simulink model "sampleModel1511"  (R2023a)
settings: Solver=VariableStepAuto  StartTime=0.0  StopTime=10.0  RelTol=1e-3
libraries: hdlsllib x6, simulink x4
settings Model: Creator=user1  LastModifiedBy=user1

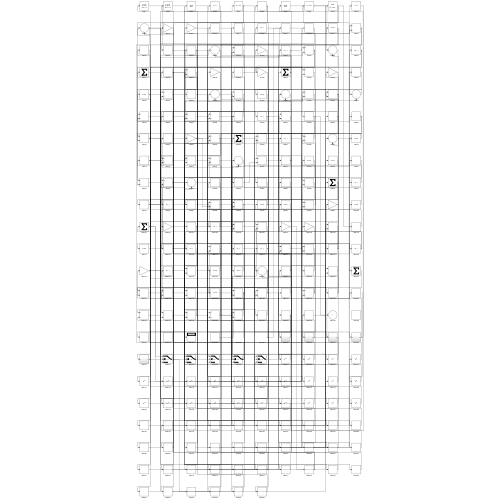
[thumbnail: Simulink's stored preview of the top-level diagram]
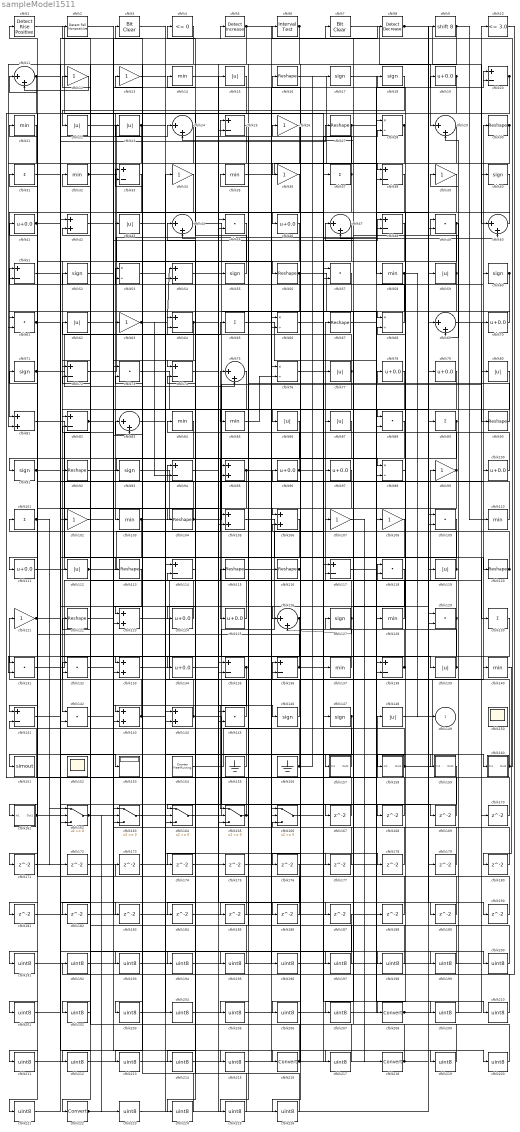
== system sampleModel1511 ==
  cfblk1 : hdlsllib/Logic and Bit Operations/Detect Rise Positive  vinit=0  OutDataTypeStr=boolean
  cfblk10 : hdlsllib/Logic and Bit Operations/Compare To Constant  relop=<=  const=3.0  OutDataTypeStr=boolean
  cfblk{19,41,46,70,78..79,96..97,100,111,124..125,134} (13 alike) : Bias  Bias=0.0  SaturateOnIntegerOverflow=off
  cfblk{31,37,65,89,101,130} (6 alike) : Sum  Inputs=+
  cfblk{12..13,26,34,36,39,63,99,102,107..108,121} (12 alike) : Gain
  cfblk{14,21,32,35,58,84..85,103,110,128,137,140} (12 alike) : MinMax
  cfblk{16,27,30,56,67,90,92,104,113,115..116,120,122} (13 alike) : Reshape
  cfblk{42,54,81,95,105..106,123,133,143..144} (10 alike) : Sum
  cfblk{45,49,57,61,73,88,109,118,129,131..132,142,145} (13 alike) : DotProduct  OutDataTypeStr=Inherit: Inherit via internal rule
  cfblk{11,24,29,44,47,50,69,75,83,126} (10 alike) : Sum  Inputs=|++
  cfblk{15,22..23,43,59,62,77,80,86..87,112,119,139,148} (14 alike) : Abs  SaturateOnIntegerOverflow=off
  cfblk{20,25,33,38,48,51,64,72,74,82,94,114,117,135..136,138,141} (17 alike) : Sum  Inputs=+-
  cfblk{17..18,40,52,55,60,71,91,93,127,146..147} (12 alike) : Signum
  cfblk150 : Scope
      settings: Floating=on
  cfblk151 : ToWorkspace  VariableName=simout  SaveFormat=Timeseries  SampleTime=-1
  cfblk152 : Scope
      settings: Floating=on
  cfblk153 : Display
  cfblk154 : hdlsllib/Sources/Counter Free-Running  NumBits=16  tsamp=-1
  cfblk155 : Ground
  cfblk156 : Ground
  cfblk157 : Subsystem
      settings: LibrarySourceBlock=|
      | hdlsllib/Ports &
      | Subsystems/Subsystem
  cfblk158 : Subsystem
      settings: LibrarySourceBlock=|
      | hdlsllib/Ports &
      | Subsystems/Subsystem
  cfblk159 : Subsystem
      settings: LibrarySourceBlock=|
      | hdlsllib/Ports &
      | Subsystems/Subsystem
  cfblk160 : Subsystem
      settings: LibrarySourceBlock=|
      | hdlsllib/Ports &
      | Subsystems/Subsystem
  cfblk161 : Subsystem
      settings: LibrarySourceBlock=|
      | hdlsllib/Ports &
      | Subsystems/Subsystem
  cfblk{162..166} (5 alike) : Switch  SaturateOnIntegerOverflow=off  InputSameDT=off
  cfblk{167..190} (24 alike) : Delay  SampleTime=1
  cfblk{191..207,209..215,217,219..221,223..226} (32 alike) : DataTypeConversion  OutDataTypeStr=uint8  SaturateOnIntegerOverflow=off  RndMeth=Floor
  cfblk2 : hdlsllib/Logic and Bit Operations/Detect Fall Nonpositive  vinit=0  OutDataTypeStr=boolean
  cfblk{208,216,218,222} (4 alike) : DataTypeConversion  SaturateOnIntegerOverflow=off  RndMeth=Floor
  cfblk{28,53,66,68,76,98} (6 alike) : Product  Inputs=*/  RndMeth=Zero  SaturateOnIntegerOverflow=on
  cfblk3 : simulink/Logic and Bit Operations/Bit Clear  iBit=0
      settings: LibrarySourceBlock=|
      | hdlsllib/Logic and Bit
      | Operations/Bit Clear
  cfblk4 : hdlsllib/Logic and Bit Operations/Compare To Zero  relop=<=  OutDataTypeStr=boolean
  cfblk5 : simulink/Logic and Bit Operations/Detect Increase  vinit=0.0  OutDataTypeStr=boolean
      settings: LibrarySourceBlock=|
      | hdlsllib/Logic and Bit
      | Operations/Detect
      | Increase
  cfblk6 : hdlsllib/Logic and Bit Operations/Interval Test  IntervalClosedRight=on  uplimit=0.5  IntervalClosedLeft=on  lowlimit=-0.5  OutDataTypeStr=boolean
  cfblk7 : simulink/Logic and Bit Operations/Bit Clear  iBit=0
      settings: LibrarySourceBlock=|
      | hdlsllib/Logic and Bit
      | Operations/Bit Clear
  cfblk8 : simulink/Logic and Bit Operations/Detect Decrease  vinit=0.0  OutDataTypeStr=boolean
      settings: LibrarySourceBlock=|
      | hdlsllib/Logic and Bit
      | Operations/Detect
      | Decrease
  cfblk9 : ArithShift  BitShiftNumber=8
  cfblk149 : Outport  VectorParamsAs1DForOutWhenUnconnected=off
  wires:
  cfblk20/1 -> cfblk103/1, cfblk164/3
  cfblk44/1 -> cfblk139/1
  cfblk18/1 -> cfblk22/1
  cfblk19/1 -> cfblk74/1, cfblk181/1
  cfblk33/1 -> cfblk81/1
  cfblk92/1 -> cfblk98/1
  cfblk87/1 -> cfblk125/1
  cfblk158/1(Out1) -> cfblk30/1, cfblk72/2
  cfblk65/1 -> cfblk138/1
  cfblk107/1 -> cfblk218/1
  cfblk26/1 -> cfblk91/1
  cfblk128/1 -> cfblk67/1
  cfblk32/1 -> cfblk56/1, cfblk72/1, cfblk215/1
  cfblk78/1 -> cfblk88/1
  cfblk123/1 -> cfblk136/1
  cfblk59/1 -> cfblk141/1, cfblk24/2, cfblk165/3
  cfblk157/1(Out1) -> cfblk83/1
  cfblk55/1 -> cfblk4/1
  cfblk84/1 -> cfblk133/1
  cfblk75/1 -> cfblk142/1
  cfblk160/1(Out1) -> cfblk6/1, cfblk33/1
  cfblk63/1 -> cfblk54/1, cfblk94/2
  cfblk15/1 -> cfblk143/1
  cfblk11/1 -> cfblk148/1, cfblk129/2, cfblk189/1
  cfblk71/1 -> cfblk64/1, cfblk75/2
  cfblk47/1 -> cfblk82/1
  cfblk159/1(Out1) -> cfblk164/1
  cfblk161/1(Out1) -> cfblk51/2, cfblk183/1
  cfblk37/1 -> cfblk14/1, cfblk162/2
  cfblk126/1 -> cfblk131/2, cfblk185/1
  cfblk60/1 -> cfblk157/1(In1), cfblk145/2
  cfblk80/1 -> cfblk158/1(In1)
  cfblk72/1 -> cfblk48/1
  cfblk46/1 -> cfblk123/1
  cfblk103/1 -> cfblk9/1, cfblk182/1
  cfblk38/1 -> cfblk106/1
  cfblk112/1 -> cfblk75/1, cfblk8/1
  cfblk85/1 -> cfblk76/2
  cfblk91/1 -> cfblk27/1, cfblk5/1, cfblk217/1
  cfblk62/1 -> cfblk216/1
  cfblk89/1 -> cfblk104/1, cfblk207/1
  cfblk129/1 -> cfblk74/2, cfblk174/1
  cfblk148/1 -> cfblk89/1
  cfblk164/1 -> cfblk37/1
  cfblk77/1 -> cfblk32/1, cfblk163/3
  cfblk23/1 -> cfblk43/1, cfblk177/1
  cfblk22/1 -> cfblk77/1
  cfblk16/1 -> cfblk58/1
  cfblk41/1 -> cfblk161/1(In1), cfblk135/2
  cfblk119/1 -> cfblk7/1, cfblk47/2
  cfblk50/1 -> cfblk46/1
  cfblk111/1 -> cfblk64/2
  cfblk35/1 -> cfblk38/1
  cfblk96/1 -> cfblk84/1, cfblk50/2
  cfblk134/1 -> cfblk15/1
  cfblk141/1 -> cfblk100/1
  cfblk110/1 -> cfblk41/1
  cfblk70/1 -> cfblk68/1
  cfblk156/1 -> cfblk94/1, cfblk17/1
  cfblk133/1 -> cfblk99/1
  cfblk136/1 -> cfblk51/1, cfblk168/1
  cfblk25/1 -> cfblk144/2
  cfblk101/1 -> cfblk162/1, cfblk172/1
  cfblk79/1 -> cfblk133/2
  cfblk146/1 -> cfblk35/1
  cfblk14/1 -> cfblk126/1
  cfblk40/1 -> cfblk44/2
  cfblk4/1 -> cfblk81/2
  cfblk143/1 -> cfblk121/1, cfblk178/1
  cfblk154/1 -> cfblk116/1
  cfblk56/1 -> cfblk128/1, cfblk134/1
  cfblk144/1 -> cfblk118/1, cfblk166/2, cfblk132/1
  cfblk3/1 -> cfblk120/1
  cfblk98/1 -> cfblk78/1
  cfblk127/1 -> cfblk126/2, cfblk12/1, cfblk3/1
  cfblk39/1 -> cfblk208/1
  cfblk116/1 -> cfblk96/1, cfblk226/1
  cfblk1/1 -> cfblk117/1
  cfblk49/1 -> cfblk112/1, cfblk69/2
  cfblk86/1 -> cfblk151/1
  cfblk125/1 -> cfblk73/2
  cfblk142/1 -> cfblk65/1
  cfblk105/1 -> cfblk147/1
  cfblk58/1 -> cfblk124/1, cfblk149/1
  cfblk131/1 -> cfblk80/1
  cfblk81/1 -> cfblk130/1
  cfblk97/1 -> cfblk113/1
  cfblk165/1 -> cfblk2/1, cfblk105/1
  cfblk29/1 -> cfblk36/1
  cfblk104/1 -> cfblk40/1, cfblk33/2
  cfblk166/1 -> cfblk137/1
  cfblk155/1 -> cfblk71/1
  cfblk64/1 -> cfblk123/2, cfblk146/1
  cfblk24/1 -> cfblk61/1
  cfblk36/1 -> cfblk54/2
  cfblk135/1 -> cfblk165/1, cfblk163/2
  cfblk163/1 -> cfblk140/1
  cfblk68/1 -> cfblk21/1
  cfblk139/1 -> cfblk18/1, cfblk29/2
  cfblk99/1 -> cfblk68/2, cfblk184/1
  cfblk9/1 -> cfblk86/1, cfblk110/1, cfblk162/3
  cfblk73/1 -> cfblk119/1
  cfblk76/1 -> cfblk28/2
  cfblk30/1 -> cfblk186/1, cfblk214/1
  cfblk120/1 -> cfblk49/1, cfblk31/1
  cfblk6/1 -> cfblk165/2, cfblk195/1
  cfblk54/1 -> cfblk118/2
  cfblk5/1 -> cfblk63/1, cfblk159/1(In1), cfblk202/1
  cfblk138/1 -> cfblk26/1, cfblk131/1
  cfblk95/1 -> cfblk20/2, cfblk211/1
  cfblk121/1 -> cfblk136/2, cfblk24/1
  cfblk106/1 -> cfblk142/2
  cfblk93/1 -> cfblk97/1
  cfblk61/1 -> cfblk105/2, cfblk193/1
  cfblk113/1 -> cfblk143/2
  cfblk124/1 -> cfblk52/1
  cfblk28/1 -> cfblk92/1, cfblk221/1
  cfblk12/1 -> cfblk11/2
  cfblk90/1 -> cfblk53/1
  cfblk117/1 -> cfblk60/1
  cfblk31/1 -> cfblk153/1
  cfblk83/1 -> cfblk160/1(In1)
  cfblk7/1 -> cfblk29/1
  cfblk21/1 -> cfblk61/2
  cfblk137/1 -> cfblk95/1
  cfblk88/1 -> cfblk111/1
  cfblk8/1 -> cfblk50/1, cfblk190/1
  cfblk145/1 -> cfblk101/1
  cfblk69/1 -> cfblk90/1
  cfblk162/1 -> cfblk48/2, cfblk223/1
  cfblk17/1 -> cfblk49/2
  cfblk34/1 -> cfblk222/1
  cfblk27/1 -> cfblk93/1, cfblk20/1
  cfblk132/1 -> cfblk19/1
  cfblk100/1 -> cfblk25/1
  cfblk82/1 -> cfblk85/1, cfblk164/2
  cfblk147/1 -> cfblk171/1, cfblk201/1
  cfblk118/1 -> cfblk167/1
  cfblk167/1 -> cfblk1/1
  cfblk168/1 -> cfblk141/2
  cfblk51/1 -> cfblk169/1
  cfblk169/1 -> cfblk47/1
  cfblk170/1 -> cfblk82/2
  cfblk171/1 -> cfblk25/2
  cfblk172/1 -> cfblk38/2
  cfblk173/1 -> cfblk88/2
  cfblk174/1 -> cfblk28/1
  cfblk74/1 -> cfblk175/1
  cfblk175/1 -> cfblk98/2
  cfblk48/1 -> cfblk176/1
  cfblk177/1 -> cfblk106/2
  cfblk178/1 -> cfblk117/2
  cfblk179/1 -> cfblk73/1
  cfblk140/1 -> cfblk180/1
  cfblk180/1 -> cfblk163/1
  cfblk181/1 -> cfblk76/1
  cfblk182/1 -> cfblk83/2
  cfblk183/1 -> cfblk138/2
  cfblk184/1 -> cfblk135/1
  cfblk185/1 -> cfblk144/1
  cfblk186/1 -> cfblk166/1
  cfblk94/1 -> cfblk187/1
  cfblk188/1 -> cfblk11/1
  cfblk189/1 -> cfblk166/3
  cfblk190/1 -> cfblk95/2
  cfblk45/1 -> cfblk191/1
  cfblk191/1 -> cfblk170/1
  cfblk10/1 -> cfblk192/1
  cfblk192/1 -> cfblk45/1
  cfblk193/1 -> cfblk45/2
  cfblk122/1 -> cfblk194/1
  cfblk194/1 -> cfblk59/1
  cfblk195/1 -> cfblk122/1
  cfblk115/1 -> cfblk196/1
  cfblk196/1 -> cfblk79/1
  cfblk2/1 -> cfblk197/1
  cfblk197/1 -> cfblk115/1
  cfblk13/1 -> cfblk198/1
  cfblk198/1 -> cfblk145/1
  cfblk43/1 -> cfblk199/1
  cfblk199/1 -> cfblk13/1
  cfblk42/1 -> cfblk200/1
  cfblk200/1 -> cfblk23/1
  cfblk201/1 -> cfblk42/1
  cfblk202/1 -> cfblk42/2
  cfblk109/1 -> cfblk203/1
  cfblk203/1 -> cfblk70/1
  cfblk53/1 -> cfblk204/1
  cfblk204/1 -> cfblk109/1
  cfblk176/1 -> cfblk205/1
  cfblk205/1 -> cfblk109/2
  cfblk108/1 -> cfblk206/1
  cfblk206/1 -> cfblk188/1
  cfblk207/1 -> cfblk108/1
  cfblk208/1 -> cfblk69/1, cfblk10/1
  cfblk67/1 -> cfblk209/1
  cfblk209/1 -> cfblk39/1
  cfblk66/1 -> cfblk210/1
  cfblk210/1 -> cfblk87/1
  cfblk211/1 -> cfblk66/1
  cfblk187/1 -> cfblk212/1
  cfblk212/1 -> cfblk66/2
  cfblk57/1 -> cfblk213/1
  cfblk213/1 -> cfblk179/1
  cfblk214/1 -> cfblk57/1
  cfblk215/1 -> cfblk57/2
  cfblk216/1 -> cfblk132/2, cfblk16/1
  cfblk217/1 -> cfblk62/1
  cfblk218/1 -> cfblk53/2, cfblk44/1
  cfblk52/1 -> cfblk219/1
  cfblk219/1 -> cfblk107/1
  cfblk102/1 -> cfblk220/1
  cfblk220/1 -> cfblk127/1
  cfblk221/1 -> cfblk102/1
  cfblk222/1 -> cfblk129/1, cfblk55/1
  cfblk223/1 -> cfblk34/1
  cfblk114/1 -> cfblk224/1
  cfblk224/1 -> cfblk173/1
  cfblk130/1 -> cfblk225/1
  cfblk225/1 -> cfblk114/1
  cfblk226/1 -> cfblk114/2

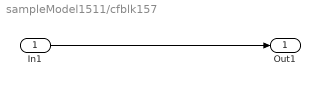
== system sampleModel1511/cfblk157 ==
  In1 : Inport
  Out1 : Outport
  wires:
  In1/1 -> Out1/1

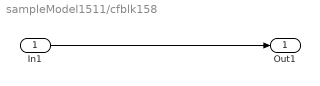
== system sampleModel1511/cfblk158 ==
  In1 : Inport
  Out1 : Outport
  wires:
  In1/1 -> Out1/1

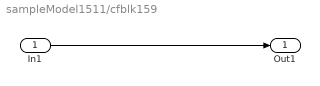
== system sampleModel1511/cfblk159 ==
  In1 : Inport
  Out1 : Outport
  wires:
  In1/1 -> Out1/1

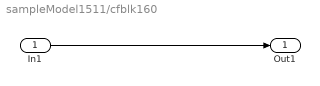
== system sampleModel1511/cfblk160 ==
  In1 : Inport
  Out1 : Outport
  wires:
  In1/1 -> Out1/1

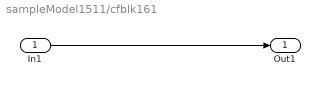
== system sampleModel1511/cfblk161 ==
  In1 : Inport
  Out1 : Outport
  wires:
  In1/1 -> Out1/1
